simulink model "auv_simulink_2018b"  (R2018b)
settings: Solver=VariableStepAuto  StartTime=0.0  StopTime=120  RelTol=1e-3
undefined symbols (not defined in the file or in its folder): B, B_buoy, Continuous, D_LIN, D_QUAD, I0, I0_buoy, m, M, M_A, M_A_buoy, m_buoy, p, r_b_b, r_b_b_buoy, r_g_b, r_g_b_buoy, T, Time
libraries: aerolibguid x2, simulink x1, cstblocks x1, ctrlSharedLib x1
settings Model: Creator=User  LastModifiedBy=Scientist
settings DataIOCC: ReturnWorkspaceOutputs=on
settings DebuggingCC: SFMachineParentedDataDiag=error

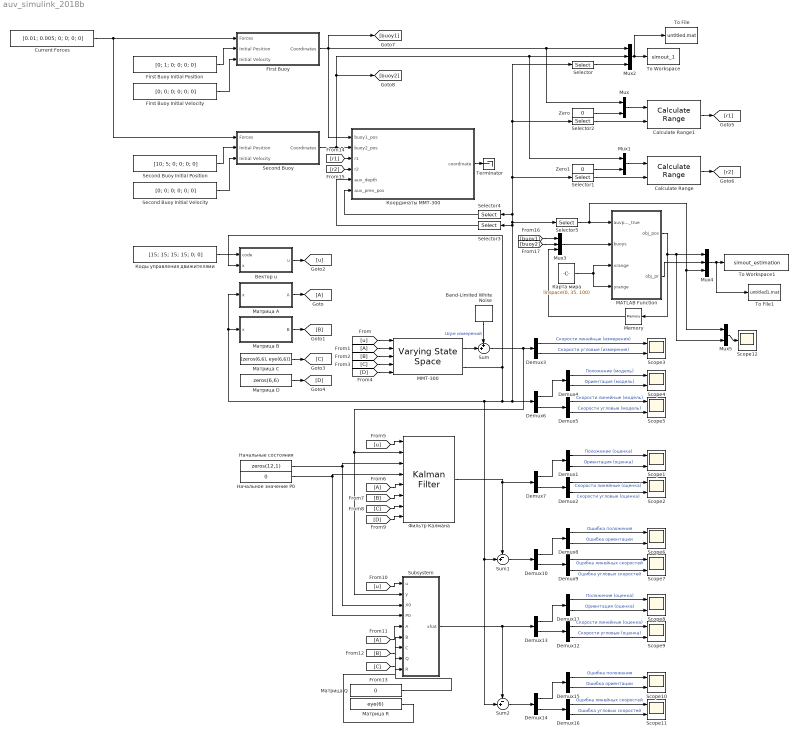
== system auv_simulink_2018b ==
  Band-Limited White Noise : simulink/Sources/Band-Limited White Noise  Cov=[0.00001]  Ts=0.1  seed=[23341]
  Calculate Range : aerolibguid/Calculate Range
      settings: SourceProductBaseCode=AE
  Calculate Range1 : aerolibguid/Calculate Range
      settings: SourceProductBaseCode=AE
  Current Forces : Constant  Value=[0.01; 0.005; 0; 0; 0; 0]
  Demux{1..16} (16 alike) : Demux  Outputs=2
  First Buoy : Subsystem
  First Buoy Initial Position : Constant  Value=[0; 1; 0; 0; 0; 0]
  First Buoy Initial Velocity : Constant  Value=[0; 0; 0; 0; 0; 0]
  MATLAB Function : MATLAB Function  TreatAsAtomicUnit=on
  MMT-300 : cstblocks/Linear Parameter Varying/Varying State Space  x0=zeros(12,1)  xNames=''  OutputX=on  OutputDX=off
  Memory : Memory  InitialCondition=[0;0]
  Mux : Mux  Inputs=2
  Mux1 : Mux  Inputs=2
  Mux2 : Mux  Inputs=3
  Mux3 : Mux  Inputs=3
  Mux4 : Mux  Inputs=3
  Mux5 : Mux  Inputs=2
  Scope{1..11} (11 alike) : Scope  NumInputPorts=2
  Scope12 : Scope
  Second Buoy : Subsystem
  Second Buoy Initial Position : Constant  Value=[10; 5; 0; 0; 0; 0]
  Second Buoy Initial Velocity : Constant  Value=[0; 0; 0; 0; 0; 0]
  Selector : Selector  InputPortWidth=12  IndexOptions=Index vector (dialog)  Indices=[1 2]  OutputSizes=1
  Selector1 : Selector  InputPortWidth=12  IndexOptions=Index vector (dialog)  Indices=[1 2 3]  OutputSizes=1
  Selector2 : Selector  InputPortWidth=12  IndexOptions=Index vector (dialog)  Indices=[1 2 3]  OutputSizes=1
  Selector3 : Selector  InputPortWidth=12  IndexOptions=Index vector (dialog)  Indices=[3]  OutputSizes=1
  Selector4 : Selector  InputPortWidth=12  IndexOptions=Index vector (dialog)  Indices=[1 2]  OutputSizes=1
  Selector5 : Selector  InputPortWidth=12  IndexOptions=Index vector (dialog)  Indices=[1 2 3]  OutputSizes=1
  Subsystem : Subsystem
  Sum : Sum  Inputs=++|
  Sum1 : Sum  Inputs=-+|
  Sum2 : Sum  Inputs=-+|
  Terminator : Terminator
  To File : ToFile  SaveFormat=Timeseries
  To File1 : ToFile  Filename=untitled1.mat  MatrixName=simout_estimation
  To Workspace : ToWorkspace  VariableName=simout_1  SaveFormat=Structure With Time  SampleTime=-1
  To Workspace1 : ToWorkspace  VariableName=simout_estimation  SaveFormat=Timeseries  SampleTime=-1
  Zero : Constant  Value=0  OutDataTypeStr=Inherit: Inherit via back propagation
  Zero1 : Constant  Value=0  OutDataTypeStr=Inherit: Inherit via back propagation
  Вектор u : MATLAB Function  TreatAsAtomicUnit=on
  Карта мира : Constant  Value=linspace(0, 35, 100)
  Коды управления движителями : Constant  Value=[15; 15; 15; 15; 0; 0]
  Координаты MMT-300 : MATLAB Function  TreatAsAtomicUnit=on
  Матрица A : MATLAB Function  TreatAsAtomicUnit=on
  Матрица B : MATLAB Function  TreatAsAtomicUnit=on
  Матрица C : Constant  Value=[zeros(6,6), eye(6,6)]
  Матрица D : Constant  Value=zeros(6,6)
  Матрица Q : Constant  Value=0
  Матрица R : Constant  Value=eye(6)
  Начальное значение P0 : Constant  Value=0
  Начальные состояния : Constant  Value=zeros(12,1)
  Фильтр Калмана : ctrlSharedLib/Kalman Filter  TimeDomain=Continuous-Time  UseCurrentEstimator=on  ModelSource=Input port  ModelSourceVariable=ss(0.95,1,1,0,1)  A=0.95  B=1  C=1  D=0  NumberOfStates=12  NumberOfInputs=6  NumberOfOutputs=6  InitialEstimateSource=Input port  X0=0  P0=10  UseK=off  UseGH=off  NumberOfProcessNoiseInputs=1  G=1  TimeInvariantG=on  H=0  TimeInvariantH=on  Q=0  TimeInvariantQ=on  R=1  TimeInvariantR=on  N=0  TimeInvariantN=on  AddInputPort=on  AddEnablePort=off  OutputEstimatedY=off  OutputP=off  Ts=-1
  wires:
  Коды управления движителями/1 -> Вектор u/1(code)
  Начальное значение P0/1 -> Subsystem/4(P0), Фильтр Калмана/4
  Demux7/1 -> Demux1/1
  Demux7/2 -> Demux2/1
  Фильтр Калмана/1 -> Demux7/1, Sum1/1
  Demux2/1 -> Scope2/1  "Скорости линейные (оценка)"
  Demux2/2 -> Scope2/2  "Скорости угловые (оценка)"
  Demux1/2 -> Scope1/2  "Ориентация (оценка)"
  Demux1/1 -> Scope1/1  "Положение (оценка)"
  Demux3/2 -> Scope3/2  "Скорости угловые (измерения)"
  Demux3/1 -> Scope3/1  "Скорости линейные (измерения)"
  Sum/1 -> Subsystem/2(y), Фильтр Калмана/2, Demux3/1
  MMT-300/1 -> Sum/2
  Band-Limited White Noise/1 -> Sum/1  "Шум измерений"
  Demux4/1 -> Scope4/1  "Положение (модель)"
  Demux4/2 -> Scope4/2  "Ориентация (модель)"
  Demux5/2 -> Scope5/2  "Скорости угловые (модель)"
  Demux5/1 -> Scope5/1  "Скорости линейные (модель)"
  Demux6/2 -> Demux5/1
  Demux6/1 -> Demux4/1
  Demux10/1 -> Demux8/1
  Demux10/2 -> Demux9/1
  Sum1/1 -> Demux10/1
  Demux9/1 -> Scope7/1  "Ошибка линейных скоростей"
  Demux9/2 -> Scope7/2  "Ошибка угловых скоростей"
  Demux8/2 -> Scope6/2  "Ошибка ориентации"
  Demux8/1 -> Scope6/1  "Ошибка положения"
  Матрица Q/1 -> Subsystem/8(Q)
  Матрица R/1 -> Subsystem/9(R)
  Demux11/1 -> Scope8/1  "Положение (оценка)"
  Demux11/2 -> Scope8/2  "Ориентация (оценка)"
  Demux12/2 -> Scope9/2  "Скорости угловые (оценка)"
  Demux12/1 -> Scope9/1  "Скорости линейные (оценка)"
  Demux13/2 -> Demux12/1
  Demux13/1 -> Demux11/1
  Матрица A/1(A) -> [A]
  Матрица B/1(B) -> [B]
  Вектор u/1(u) -> [u]
  Матрица C/1 -> [C]
  Матрица D/1 -> [D]
  [u] -> MMT-300/1
  [A] -> MMT-300/2
  [B] -> MMT-300/3
  [C] -> MMT-300/4
  [D] -> MMT-300/5
  [u] -> Фильтр Калмана/1
  [A] -> Фильтр Калмана/5
  [B] -> Фильтр Калмана/6
  [C] -> Фильтр Калмана/7
  [D] -> Фильтр Калмана/8
  [u] -> Subsystem/1(u)
  Начальные состояния/1 -> Subsystem/3(X0), Фильтр Калмана/3
  [A] -> Subsystem/5(A)
  [B] -> Subsystem/6(B)
  [C] -> Subsystem/7(C)
  Current Forces/1 -> Second Buoy/1(Forces), First Buoy/1(Forces)
  First Buoy Initial Position/1 -> First Buoy/2(Initial Position)
  First Buoy Initial Velocity/1 -> First Buoy/3(Initial Velocity)
  Second Buoy/1(Coordinates) -> [buoy2], Mux2/2, Mux1/1, Координаты MMT-300/2(buoy2_pos)
  Second Buoy Initial Velocity/1 -> Second Buoy/3(Initial Velocity)
  Second Buoy Initial Position/1 -> Second Buoy/2(Initial Position)
  First Buoy/1(Coordinates) -> [buoy1], Координаты MMT-300/1(buoy1_pos), Mux2/1, Mux/1
  Demux15/1 -> Scope10/1  "Ошибка положения"
  Demux15/2 -> Scope10/2  "Ошибка ориентации"
  Demux16/2 -> Scope11/2  "Ошибка угловых скоростей"
  Demux16/1 -> Scope11/1  "Ошибка линейных скоростей"
  Sum2/1 -> Demux14/1
  Demux14/2 -> Demux16/1
  Demux14/1 -> Demux15/1
  Subsystem/1(xhat) -> Demux13/1, Sum2/1
  Selector/1 -> Mux2/3
  MMT-300/2 -> Selector5/1, Selector2/1, Selector/1, Selector1/1, Selector4/1, Selector3/1, Demux6/1, Sum2/2, Sum1/2, Матрица A/1(x), Матрица B/1(x), Вектор u/2(x)
  Calculate Range/1 -> [r2]
  Selector2/1 -> Calculate Range1/2
  Selector3/1 -> Координаты MMT-300/5(auv_depth)
  Selector4/1 -> Координаты MMT-300/6(auv_prev_pos)
  Calculate Range1/1 -> [r1]
  Mux/1 -> Calculate Range1/1
  Zero/1 -> Mux/2
  Mux1/1 -> Calculate Range/1
  Zero1/1 -> Mux1/2
  [r1] -> Координаты MMT-300/3(r1)
  [r2] -> Координаты MMT-300/4(r2)
  Mux2/1 -> To File/1, To Workspace/1
  Координаты MMT-300/1(coordinate) -> Terminator/1
  Карта мира/1 -> MATLAB Function/3(xrange), MATLAB Function/4(yrange)
  Selector1/1 -> Calculate Range/2
  Selector5/1 -> Mux5/1, Mux4/3, MATLAB Function/1(auvpos_true)
  Mux3/1 -> MATLAB Function/2(buoys)
  [buoy1] -> Mux3/1
  [buoy2] -> Mux3/2
  MATLAB Function/1(obj_pos) -> Mux5/2, Mux4/1, Memory/1
  Memory/1 -> Mux3/3
  Mux4/1 -> To File1/1, To Workspace1/1
  MATLAB Function/2(obj_pr) -> Mux4/2
  Mux5/1 -> Scope12/1

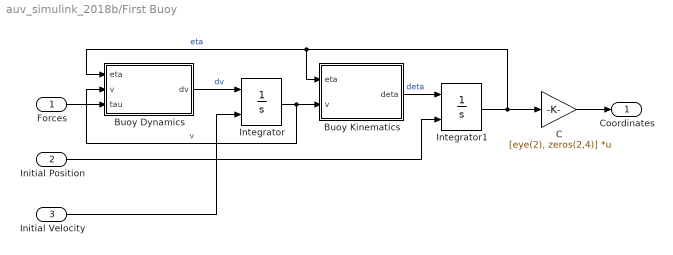
== system auv_simulink_2018b/First Buoy ==
  Forces : Inport
  Initial Position : Inport  Port=2
  Initial Velocity : Inport  Port=3
  Buoy Dynamics : MATLAB Function  TreatAsAtomicUnit=on
  Buoy Kinematics : MATLAB Function  TreatAsAtomicUnit=on
  C : Gain  Gain=[eye(2), zeros(2,4)]  Multiplication=Matrix(K*u)
  Integrator : Integrator  InitialConditionSource=external
  Integrator1 : Integrator  InitialConditionSource=external
  Coordinates : Outport  VectorParamsAs1DForOutWhenUnconnected=on
  wires:
  Buoy Dynamics/1(dv) -> Integrator/1  "dv"
  Buoy Kinematics/1(deta) -> Integrator1/1  "deta"
  C/1 -> Coordinates/1
  Integrator1/1 -> C/1, Buoy Dynamics/1(eta), Buoy Kinematics/1(eta)  "eta"
  Forces/1 -> Buoy Dynamics/3(tau)
  Integrator/1 -> Buoy Dynamics/2(v), Buoy Kinematics/2(v)  "v"
  Initial Position/1 -> Integrator1/2
  Initial Velocity/1 -> Integrator/2

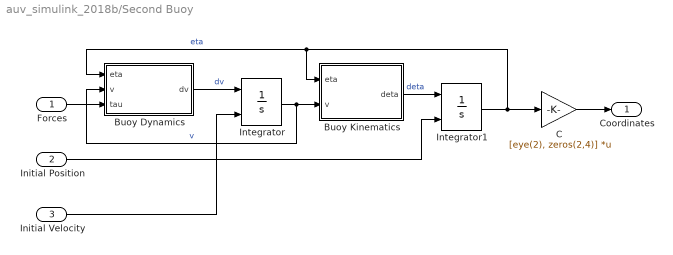
== system auv_simulink_2018b/Second Buoy ==
  Forces : Inport
  Initial Position : Inport  Port=2
  Initial Velocity : Inport  Port=3
  Buoy Dynamics : MATLAB Function  TreatAsAtomicUnit=on
  Buoy Kinematics : MATLAB Function  TreatAsAtomicUnit=on
  C : Gain  Gain=[eye(2), zeros(2,4)]  Multiplication=Matrix(K*u)
  Integrator : Integrator  InitialConditionSource=external
  Integrator1 : Integrator  InitialConditionSource=external
  Coordinates : Outport  VectorParamsAs1DForOutWhenUnconnected=on
  wires:
  Integrator/1 -> Buoy Kinematics/2(v), Buoy Dynamics/2(v)  "v"
  Forces/1 -> Buoy Dynamics/3(tau)
  Integrator1/1 -> Buoy Kinematics/1(eta), Buoy Dynamics/1(eta), C/1  "eta"
  C/1 -> Coordinates/1
  Buoy Kinematics/1(deta) -> Integrator1/1  "deta"
  Buoy Dynamics/1(dv) -> Integrator/1  "dv"
  Initial Position/1 -> Integrator1/2
  Initial Velocity/1 -> Integrator/2

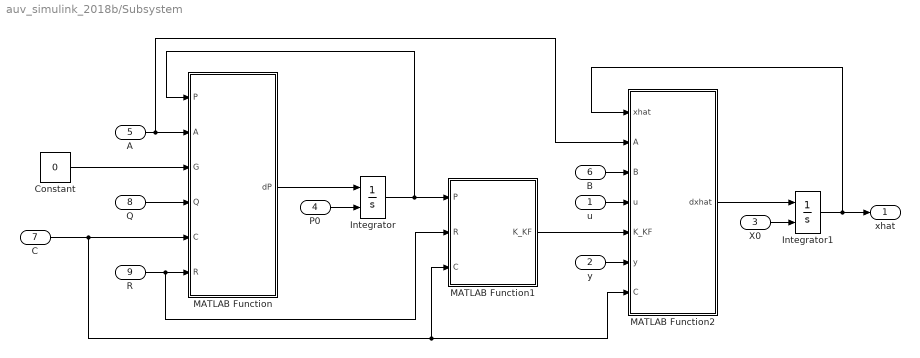
== system auv_simulink_2018b/Subsystem ==
  u : Inport
  y : Inport  Port=2
  X0 : Inport  Port=3
  P0 : Inport  Port=4
  A : Inport  Port=5
  B : Inport  Port=6
  C : Inport  Port=7
  Q : Inport  Port=8
  R : Inport  Port=9
  Constant : Constant  Value=0
  Integrator : Integrator  InitialConditionSource=external
  Integrator1 : Integrator  InitialConditionSource=external
  MATLAB Function : MATLAB Function  TreatAsAtomicUnit=on
  MATLAB Function1 : MATLAB Function  TreatAsAtomicUnit=on
  MATLAB Function2 : MATLAB Function  TreatAsAtomicUnit=on
  xhat : Outport  VectorParamsAs1DForOutWhenUnconnected=on
  wires:
  MATLAB Function/1(dP) -> Integrator/1
  P0/1 -> Integrator/2
  Integrator/1 -> MATLAB Function1/1(P), MATLAB Function/1(P)
  A/1 -> MATLAB Function2/2(A), MATLAB Function/2(A)
  Q/1 -> MATLAB Function/4(Q)
  R/1 -> MATLAB Function1/2(R), MATLAB Function/6(R)
  C/1 -> MATLAB Function2/7(C), MATLAB Function1/3(C), MATLAB Function/5(C)
  MATLAB Function2/1(dxhat) -> Integrator1/1
  X0/1 -> Integrator1/2
  MATLAB Function1/1(K_KF) -> MATLAB Function2/5(K_KF)
  Integrator1/1 -> MATLAB Function2/1(xhat), xhat/1
  B/1 -> MATLAB Function2/3(B)
  u/1 -> MATLAB Function2/4(u)
  y/1 -> MATLAB Function2/6(y)
  Constant/1 -> MATLAB Function/3(G)

== matlab function auv_simulink_2018b/Subsystem/MATLAB Function1 ==
  data: P input; R input; K_KF output; C input
function K_KF = FilterGain(P,R,C)
K_KF = P*C'*inv(R);

== matlab function auv_simulink_2018b/Subsystem/MATLAB Function ==
  data: P input; A input; dP output; G input; Q input; C input; R input
function dP = DerivativeP(P,A,G,Q,C,R)
G = eye(length(Q));
dP = A*P + P*A' + G*Q*G' - P*C'*inv(R)*C*P;

== matlab function auv_simulink_2018b/Матрица A ==
  data: x input size=12; A output size=[12 12]; M parameter; I0 parameter; r_g_b parameter; m parameter; r_b_b parameter; M_A parameter; D_LIN parameter; D_QUAD parameter
function A = Matrix_A(x, M, I0, r_g_b, m, r_b_b, M_A, D_LIN, D_QUAD)
n = 6;
eta = x(1:n); 
v = x(7:end);

%% ВСПОМОГАТЕЛЬНЫЕ ФУНКЦИИ
% преобразование в кососимметричную матрицу
S = @(x)([ 0 -x(3) x(2); x(3) 0 -x(1); -x(2) x(1) 0 ]); 

%% РАСЧЕТ ЯКОБИАНА
J_k_o = @(eta)[ 1  0           -sin(eta(5)); ...
                0  cos(eta(4))  cos(eta(5))*sin(eta(4)); ...
                0 -sin(eta(4))  cos(eta(5))*cos(eta(4)) ];
R_I_B = @(eta)[ cos(eta(6))*cos(eta(5))                                        sin(eta(6))*cos(eta(5))                                       -sin(eta(5)); ...
               -sin(eta(6))*cos(eta(4)) + cos(eta(6))*sin(eta(5))*sin(eta(4))  cos(eta(6))*cos(eta(4)) + sin(eta(6))*sin(eta(5))*sin(eta(4))  sin(eta(4))*cos(eta(5)); ...
                sin(eta(6))*sin(eta(4)) + cos(eta(6))*sin(eta(5))*cos(eta(4)) -cos(eta(6))*sin(eta(4)) + sin(eta(6))*sin(eta(5))*cos(eta(4))  cos(eta(4))*cos(eta(5)) ];
J = @(eta)[ R_I_B(eta) zeros(3); ...
            zeros(3)   J_k_o(eta) ];

%% РАСЧЕТ C(v)
% расчет C_RB(v)
%C_RB = @(v)([ zeros(3) -m*S(v(1:3)); -m*S(v(1:3)) -S(diag(I0).*v(4:end)) ]); 
C_RB = @(v)[ zeros(3)                           -m*S(v(1:3))-m*S(S(v(4:end))*r_g_b); ...
            -m*S(v(1:3))-m*S(S(v(4:end))*r_g_b)  m*S(S(v(1:3))*r_g_b)-S(I0*v(4:end)) ];
% расчет C_A(v)
diag_M_A = diag(M_A);
C_A = @(v)([ zeros(3) -S(diag_M_A(1:3).*v(1:3));
    -S(diag_M_A(1:3).*v(1:3)) -S(diag_M_A(4:end).*v(4:end))]);
% расчет C(v)
C = @(v)(C_RB(v) + C_A(v)); 
% M11 = M(1:3,1:3); M12 = M(1:3,4:6); M21 = M(4:6,1:3); M22 = M(4:6,4:6);
% C = @(v)[ zeros(3) -S(M11*v(1:3)+M12*v(4:6)); -S(M11*v(1:3)+M12*v(4:6)) -S(M21*v(1:3)+M22*v(4:6)) ];

%% РАСЧЕТ D(v)
D = @(v)(D_LIN + D_QUAD.*diag(abs(v))); 

A = [zeros(n), J(eta)^-1;
     zeros(n), -M^-1 * ( C(v) + D(v) )];

== matlab function auv_simulink_2018b/Матрица B ==
  data: x input size=12; B output size=[12 6]; M parameter
function B = Matrix_B(x, M)
n = 6;
B = [zeros(n); M^-1];

== matlab function auv_simulink_2018b/Вектор u ==
  data: code input [-127..127]; x input size=12; u output size=6; T parameter; p parameter; B parameter; m parameter; r_g_b parameter; r_b_b parameter
function u = Vector_u(code,x, T, p, B, m, r_g_b, r_b_b)
n = 6;
eta = x(1:n); 

%% РАСЧЕТ g(n)
x_g = r_g_b(1); y_g = r_g_b(2); z_g = r_g_b(3);
x_b = r_b_b(1); y_b = r_b_b(2); z_b = r_b_b(3);
g = @(eta)[ (m*9.81-B)*sin(eta(5)); 
           -(m*9.81-B)*cos(eta(5))*sin(eta(4)); 
           -(m*9.81-B)*cos(eta(5))*cos(eta(4));
           -(y_g*m*9.81-y_b*B)*cos(eta(5))*cos(eta(4)) + ...
              (z_g*m*9.81-z_b*B)*cos(eta(5))*sin(eta(4));
            (z_g*m*9.81-z_b*B)*sin(eta(5)) + ...
              (x_g*m*9.81-x_b*B)*cos(eta(5))*cos(eta(4));
           -(x_g*m*9.81-x_b*B)*cos(eta(5))*sin(eta(4)) - ...
              (y_g*m*9.81-y_b*B)*sin(eta(5)) ]; 


F = @(code)polyval(p,code);

f1 = @(code)[ F(code)*cos(deg2rad(22)); 
              0; 
              F(code)*sin(deg2rad(22)) ];
f2 = @(code)[ F(code)*cos(deg2rad(22)); 
              F(code)*sin(deg2rad(22));
              0 ];
f3 = @(code)[ F(code)*cos(deg2rad(22)); 
              0; 
              -F(code)*sin(deg2rad(22)) ];
f4 = @(code)[ F(code)*cos(deg2rad(22));  
              -F(code)*sin(deg2rad(22));
              0 ];
f5 = @(code)[ 0; 
              F(code); 
              0 ];
f6 = @(code)[ 0; 
              0; 
              -F(code) ];

r1 = T(1,:)'; 
r2 = T(2,:)'; 
r3 = T(3,:)';
r4 = T(4,:)';
r5 = T(5,:)';
r6 = T(6,:)';
tau1 = @(code)[ f1(code); cross(r1, f1(code)) ];
tau2 = @(code)[ f2(code); cross(r2, f2(code)) ];
tau3 = @(code)[ f3(code); cross(r3, f3(code)) ];
tau4 = @(code)[ f4(code); cross(r4, f4(code)) ];
tau5 = @(code)[ f5(code); cross(r5, f5(code)) ];
tau6 = @(code)[ f6(code); cross(r6, f6(code)) ];

tau_c = @(code)[ tau1(code(1)), tau2(code(2)), tau3(code(3)), ...
                 tau4(code(4)), tau5(code(5)), tau6(code(6)) ];

thruster_mask = [1, 1, 1, 1, 1, 1]';

u = -g(eta) + tau_c(code) * thruster_mask;

== matlab function auv_simulink_2018b/Subsystem/MATLAB Function2 ==
  data: xhat input; A input; B input; dxhat output; u input; K_KF input; y input; C input
function dxhat = Derivative_xhat(xhat,A,B,u,K_KF,y,C)
dxhat = A*xhat + B*u + K_KF*(y - C*xhat);

== matlab function auv_simulink_2018b/First Buoy/Buoy Dynamics ==
  data: eta input; dv output; v input; tau input; m_buoy parameter; r_g_b_buoy parameter; r_b_b_buoy parameter; I0_buoy parameter; M_A_buoy parameter size=[6 6]; B_buoy parameter
function dv = Dynamics(eta, v, tau, m_buoy, r_g_b_buoy, r_b_b_buoy, I0_buoy, M_A_buoy, B_buoy)

%% ВСПОМОГАТЕЛЬНЫЕ ФУНКЦИИ
% преобразование в кососимметричную матрицу
S = @(x)([ 0 -x(3) x(2); x(3) 0 -x(1); -x(2) x(1) 0 ]); 

%% РАСЧЕТ ЯКОБИАНА
J_k_o = @(eta)[ 1  0           -sin(eta(5)); ...
                0  cos(eta(4))  cos(eta(5))*sin(eta(4)); ...
                0 -sin(eta(4))  cos(eta(5))*cos(eta(4)) ];
R_I_B = @(eta)[ cos(eta(6))*cos(eta(5))                                        sin(eta(6))*cos(eta(5))                                       -sin(eta(5)); ...
               -sin(eta(6))*cos(eta(4)) + cos(eta(6))*sin(eta(5))*sin(eta(4))  cos(eta(6))*cos(eta(4)) + sin(eta(6))*sin(eta(5))*sin(eta(4))  sin(eta(4))*cos(eta(5)); ...
                sin(eta(6))*sin(eta(4)) + cos(eta(6))*sin(eta(5))*cos(eta(4)) -cos(eta(6))*sin(eta(4)) + sin(eta(6))*sin(eta(5))*cos(eta(4))  cos(eta(4))*cos(eta(5)) ];
J = @(eta)[ R_I_B(eta) zeros(3); ...
            zeros(3)   J_k_o(eta) ];

%% РАСЧЕТ МАТРИЦЫ M
% расчет M_RB
M_RB_buoy = [ m_buoy*eye(3) -m_buoy*S(r_g_b_buoy); m_buoy*S(r_g_b_buoy) I0_buoy ]; 
% расчет M
M_buoy = M_RB_buoy + M_A_buoy; 

%% РАСЧЕТ C(v)
% расчет C_RB(v)
%C_RB = @(v)([ zeros(3) -m*S(v(1:3)); -m*S(v(1:3)) -S(diag(I0).*v(4:end)) ]); 
C_RB_buoy = @(v)[ zeros(3)                           -m_buoy*S(v(1:3))-m_buoy*S(S(v(4:end))*r_g_b_buoy); ...
                 -m_buoy*S(v(1:3))-m_buoy*S(S(v(4:end))*r_g_b_buoy)  m_buoy*S(S(v(1:3))*r_g_b_buoy)-S(I0_buoy*v(4:end)) ];
% расчет C_A(v)
diag_M_A_buoy = diag(M_A_buoy);
C_A_buoy = @(v)([ zeros(3) -S(diag_M_A_buoy(1:3).*v(1:3)); 
    -S(diag_M_A_buoy(1:3).*v(1:3)) -S(diag_M_A_buoy(4:end).*v(4:end))]);
% расчет C(v)
C_buoy = @(v)(C_RB_buoy(v) + C_A_buoy(v)); 

%% РАСЧЕТ D(v)
D_buoy = @(v)(eye(6)); 

%% РАСЧЕТ g(n)
x_g_buoy = r_g_b_buoy(1); y_g_buoy = r_g_b_buoy(2); z_g_buoy = r_g_b_buoy(3);
x_b_buoy = r_b_b_buoy(1); y_b_buoy = r_b_b_buoy(2); z_b_buoy = r_b_b_buoy(3);
g_buoy = @(eta)[ (m_buoy*9.81-B_buoy)*sin(eta(5)); 
           -(m_buoy*9.81-B_buoy)*cos(eta(5))*sin(eta(4)); 
           -(m_buoy*9.81-B_buoy)*cos(eta(5))*cos(eta(4));
           -(y_g_buoy*m_buoy*9.81-y_b_buoy*B_buoy)*cos(eta(5))*cos(eta(4)) + ...
              (z_g_buoy*m_buoy*9.81-z_b_buoy*B_buoy)*cos(eta(5))*sin(eta(4));
            (z_g_buoy*m_buoy*9.81-z_b_buoy*B_buoy)*sin(eta(5)) + ...
              (x_g_buoy*m_buoy*9.81-x_b_buoy*B_buoy)*cos(eta(5))*cos(eta(4));
           -(x_g_buoy*m_buoy*9.81-x_b_buoy*B_buoy)*cos(eta(5))*sin(eta(4)) - ...
              (y_g_buoy*m_buoy*9.81-y_b_buoy*B_buoy)*sin(eta(5)) ]; 

dv = -M_buoy^-1 * ( C_buoy(v)*v + D_buoy(v)*v + g_buoy(eta) - J(eta)'*tau );

== matlab function auv_simulink_2018b/First Buoy/Buoy Kinematics ==
  data: eta input; v input; deta output
function deta = Kinematics(eta, v)
%% ВСПОМОГАТЕЛЬНЫЕ ФУНКЦИИ
% преобразование в кососимметричную матрицу
S = @(x)([ 0 -x(3) x(2); x(3) 0 -x(1); -x(2) x(1) 0 ]); 

%% РАСЧЕТ ЯКОБИАНА
J_k_o = @(eta)[ 1  0           -sin(eta(5)); ...
                0  cos(eta(4))  cos(eta(5))*sin(eta(4)); ...
                0 -sin(eta(4))  cos(eta(5))*cos(eta(4)) ];
R_I_B = @(eta)[ cos(eta(6))*cos(eta(5))                                        sin(eta(6))*cos(eta(5))                                       -sin(eta(5)); ...
               -sin(eta(6))*cos(eta(4)) + cos(eta(6))*sin(eta(5))*sin(eta(4))  cos(eta(6))*cos(eta(4)) + sin(eta(6))*sin(eta(5))*sin(eta(4))  sin(eta(4))*cos(eta(5)); ...
                sin(eta(6))*sin(eta(4)) + cos(eta(6))*sin(eta(5))*cos(eta(4)) -cos(eta(6))*sin(eta(4)) + sin(eta(6))*sin(eta(5))*cos(eta(4))  cos(eta(4))*cos(eta(5)) ];
J = @(eta)[ R_I_B(eta) zeros(3); ...
            zeros(3)   J_k_o(eta) ];
deta = J(eta)^-1 * v;

== matlab function auv_simulink_2018b/Second Buoy/Buoy Dynamics ==
  data: eta input; dv output; v input; tau input; m_buoy parameter; r_g_b_buoy parameter; r_b_b_buoy parameter; I0_buoy parameter; M_A_buoy parameter size=[6 6]; B_buoy parameter
function dv = Dynamics(eta, v, tau, m_buoy, r_g_b_buoy, r_b_b_buoy, I0_buoy, M_A_buoy, B_buoy)

%% ВСПОМОГАТЕЛЬНЫЕ ФУНКЦИИ
% преобразование в кососимметричную матрицу
S = @(x)([ 0 -x(3) x(2); x(3) 0 -x(1); -x(2) x(1) 0 ]); 

%% РАСЧЕТ ЯКОБИАНА
J_k_o = @(eta)[ 1  0           -sin(eta(5)); ...
                0  cos(eta(4))  cos(eta(5))*sin(eta(4)); ...
                0 -sin(eta(4))  cos(eta(5))*cos(eta(4)) ];
R_I_B = @(eta)[ cos(eta(6))*cos(eta(5))                                        sin(eta(6))*cos(eta(5))                                       -sin(eta(5)); ...
               -sin(eta(6))*cos(eta(4)) + cos(eta(6))*sin(eta(5))*sin(eta(4))  cos(eta(6))*cos(eta(4)) + sin(eta(6))*sin(eta(5))*sin(eta(4))  sin(eta(4))*cos(eta(5)); ...
                sin(eta(6))*sin(eta(4)) + cos(eta(6))*sin(eta(5))*cos(eta(4)) -cos(eta(6))*sin(eta(4)) + sin(eta(6))*sin(eta(5))*cos(eta(4))  cos(eta(4))*cos(eta(5)) ];
J = @(eta)[ R_I_B(eta) zeros(3); ...
            zeros(3)   J_k_o(eta) ];

%% РАСЧЕТ МАТРИЦЫ M
% расчет M_RB
M_RB_buoy = [ m_buoy*eye(3) -m_buoy*S(r_g_b_buoy); m_buoy*S(r_g_b_buoy) I0_buoy ]; 
% расчет M
M_buoy = M_RB_buoy + M_A_buoy; 

%% РАСЧЕТ C(v)
% расчет C_RB(v)
%C_RB = @(v)([ zeros(3) -m*S(v(1:3)); -m*S(v(1:3)) -S(diag(I0).*v(4:end)) ]); 
C_RB_buoy = @(v)[ zeros(3)                           -m_buoy*S(v(1:3))-m_buoy*S(S(v(4:end))*r_g_b_buoy); ...
                 -m_buoy*S(v(1:3))-m_buoy*S(S(v(4:end))*r_g_b_buoy)  m_buoy*S(S(v(1:3))*r_g_b_buoy)-S(I0_buoy*v(4:end)) ];
% расчет C_A(v)
diag_M_A_buoy = diag(M_A_buoy);
C_A_buoy = @(v)([ zeros(3) -S(diag_M_A_buoy(1:3).*v(1:3)); 
    -S(diag_M_A_buoy(1:3).*v(1:3)) -S(diag_M_A_buoy(4:end).*v(4:end))]);
% расчет C(v)
C_buoy = @(v)(C_RB_buoy(v) + C_A_buoy(v)); 

%% РАСЧЕТ D(v)
D_buoy = @(v)(eye(6)); 

%% РАСЧЕТ g(n)
x_g_buoy = r_g_b_buoy(1); y_g_buoy = r_g_b_buoy(2); z_g_buoy = r_g_b_buoy(3);
x_b_buoy = r_b_b_buoy(1); y_b_buoy = r_b_b_buoy(2); z_b_buoy = r_b_b_buoy(3);
g_buoy = @(eta)[ (m_buoy*9.81-B_buoy)*sin(eta(5)); 
           -(m_buoy*9.81-B_buoy)*cos(eta(5))*sin(eta(4)); 
           -(m_buoy*9.81-B_buoy)*cos(eta(5))*cos(eta(4));
           -(y_g_buoy*m_buoy*9.81-y_b_buoy*B_buoy)*cos(eta(5))*cos(eta(4)) + ...
              (z_g_buoy*m_buoy*9.81-z_b_buoy*B_buoy)*cos(eta(5))*sin(eta(4));
            (z_g_buoy*m_buoy*9.81-z_b_buoy*B_buoy)*sin(eta(5)) + ...
              (x_g_buoy*m_buoy*9.81-x_b_buoy*B_buoy)*cos(eta(5))*cos(eta(4));
           -(x_g_buoy*m_buoy*9.81-x_b_buoy*B_buoy)*cos(eta(5))*sin(eta(4)) - ...
              (y_g_buoy*m_buoy*9.81-y_b_buoy*B_buoy)*sin(eta(5)) ]; 

dv = -M_buoy^-1 * ( C_buoy(v)*v + D_buoy(v)*v + g_buoy(eta) - J(eta)'*tau );

== matlab function auv_simulink_2018b/Second Buoy/Buoy Kinematics ==
  data: eta input; v input; deta output
function deta = Kinematics(eta, v)
%% ВСПОМОГАТЕЛЬНЫЕ ФУНКЦИИ
% преобразование в кососимметричную матрицу
S = @(x)([ 0 -x(3) x(2); x(3) 0 -x(1); -x(2) x(1) 0 ]); 

%% РАСЧЕТ ЯКОБИАНА
J_k_o = @(eta)[ 1  0           -sin(eta(5)); ...
                0  cos(eta(4))  cos(eta(5))*sin(eta(4)); ...
                0 -sin(eta(4))  cos(eta(5))*cos(eta(4)) ];
R_I_B = @(eta)[ cos(eta(6))*cos(eta(5))                                        sin(eta(6))*cos(eta(5))                                       -sin(eta(5)); ...
               -sin(eta(6))*cos(eta(4)) + cos(eta(6))*sin(eta(5))*sin(eta(4))  cos(eta(6))*cos(eta(4)) + sin(eta(6))*sin(eta(5))*sin(eta(4))  sin(eta(4))*cos(eta(5)); ...
                sin(eta(6))*sin(eta(4)) + cos(eta(6))*sin(eta(5))*cos(eta(4)) -cos(eta(6))*sin(eta(4)) + sin(eta(6))*sin(eta(5))*cos(eta(4))  cos(eta(4))*cos(eta(5)) ];
J = @(eta)[ R_I_B(eta) zeros(3); ...
            zeros(3)   J_k_o(eta) ];
deta = J(eta)^-1 * v;

== matlab function auv_simulink_2018b/Координаты MMT-300 ==
  data: buoy1_pos input size=2 [-127..127]; buoy2_pos input size=2; r1 input size=1; r2 input size=1; coordinate output size=2; auv_depth input size=1; auv_prev_pos input size=2
function coordinate = Compute_Coordinates(buoy1_pos, buoy2_pos, r1, r2, auv_depth, auv_prev_pos)
x_b1 = buoy1_pos(1); y_b1 = buoy1_pos(2); z_b1 = 0;
x_b2 = buoy2_pos(1); y_b2 = buoy2_pos(2); z_b2 = 0;

%% https://stackoverflow.com/questions/5238566/intersection-points-of-two-circles-in-matlab

A = [x_b1 y_b1]; %# center of the first circle
B = [x_b2 y_b2]; %# center of the second circle
a = sqrt(r2^2 - auv_depth^2); %# radius of the SECOND circle
b = sqrt(r1^2 - auv_depth^2); %# radius of the FIRST circle
c = norm(A-B); %# distance between circles

cosAlpha = (b^2+c^2-a^2)/(2*b*c);

u_AB = (B - A)/c; %# unit vector from first to second center
pu_AB = [u_AB(2), -u_AB(1)]; %# perpendicular vector to unit vector

%# use the cosine of alpha to calculate the length of the
%# vector along and perpendicular to AB that leads to the
%# intersection point
intersect_1 = A + u_AB * (b*cosAlpha) + pu_AB * (b*sqrt(1-cosAlpha^2));
intersect_2 = A + u_AB * (b*cosAlpha) - pu_AB * (b*sqrt(1-cosAlpha^2));


norm_est = [ norm([intersect_1(1) - auv_prev_pos(1), intersect_1(2) - auv_prev_pos(2)], 2); ...
             norm([intersect_2(1) - auv_prev_pos(1), intersect_2(2) - auv_prev_pos(2)], 2) ];

[~, idx] = min(norm_est);

if idx==1
    coordinate = intersect_1';
else
    coordinate = intersect_2';
end

== matlab function auv_simulink_2018b/MATLAB Function ==
  data: obj_pos output; auvpos_true input; obj_pr output; buoys input; xrange input; yrange input
%%
% Возвращает наиболее вероятное положение аппарата в зависимости от
% распределения и его параметров.
function [obj_pos, obj_pr]  = getMostProbPos(auvpos_true, buoys, xrange, yrange)
auvpos_true = auvpos_true(1:2);
buoys = reshape(buoys, 2, 3);
buoys_len = 3;

allDtb = ones(length(xrange), length(yrange)); 

% Вероятности местонахождения на фазовой плоскости для каждого буя
for i = 1:buoys_len
%     buoys(i).dtb = [];   % prob. distribution
    pos = buoys(:,i);   % [x,y] - position
    d = getDist(auvpos_true, pos);   % Действительное расстояние до аппарата
    Nx0 = [0 0.5];

    dtb = zeros(length(xrange)*length(yrange),1);
    for k = 1:length(xrange)
        x = xrange(k);
        for j = 1:length(yrange)
            y = yrange(j);
            dtb((k-1)*length(yrange)+j) = prDstFun(getDist(pos, [x;y]), d(1) + Nx0(1), Nx0(2));
        end
    end    

    dtb = reshape(dtb, length(xrange), length(yrange));
    
    allDtb = allDtb .* dtb;
end

% i=1;
% j=1;
% obj_pr = max(allDtb, [], 'all', 'omitnan');
% obj_pr = max(max(allDtb));
obj_pr = max(max(allDtb));
% [i,j] = find(allDtb == obj_pr);

stop = 0;
for i = 1:length(xrange)
    for j = 1:length(yrange)
        if (allDtb(i,j) == obj_pr)
            stop = 1;
            break
        end
    end
    if stop == 1
        break
    end
end

obj_pos = [xrange(j); yrange(i)];
end



%% PDF for normal distribution
function pdf_o = prDstFun(x, mu, sig)
pdf_o = exp(-0.5*(x-mu)^2/(sig^2)) / (sig*sqrt(2*pi));
% pdf_o = pdf('Normal',x, mu, sig);   % супер медленно
end



%% Distance between points A and B
function d = getDist(a,b)
%     d = sqrt((a(1)-b(1))^2+(a(2)-b(2))^2);
d = norm(b-a);
end
